simulink model "STM_sim"  (R2024b)
settings: Solver=ode3  StartTime=0.0  StopTime=time_simulated  FixedStep=time_step_size  RelTol=1e-3
values from neighbouring files (symbols this model uses):
  a = 0.276626506024    [Fufy.mat]    (also in STMDrift.m = 1.347; Trajectory_LQR_double_track_Workspace_Phase_Plane_16_06.m = l-b; initParam.m = l-b)
  b = 0.283373493976    [Fufy.mat]    (also in STMDrift.m = 1.393; Trajectory_LQR_double_track_Workspace_Phase_Plane_16_06.m = l/2; initParam.m = l/2)
  constant_force = 9    [runSIM.m]
  constant_steer = deg2rad(15)    [runSIM.m]
  Fz_Front_nominal = Fz_Front    [initParam.m]
  Fz_Rear_nominal = Fz_Rear    [initParam.m]
  gamma = pi/2    (= 1.57079632679)    [Trajectory_LQR_double_track_Workspace_Phase_Plane_16_06.m]    (also in initParam.m)
  J_CoG = 1.30125108434    [Fufy.mat]    (also in Trajectory_LQR_double_track_Workspace_Phase_Plane_16_06.m = 9.4*a^2+9.4*b^2; initParam.m = 9.4*a^2+9.4*b^2)
  m = 16.6    [Fufy.mat]    (also in STMDrift.m = 2137.3; Trajectory_LQR_double_track_Workspace_Phase_Plane_16_06.m = 18.8; initParam.m = 18.8)
  steering_ratio_f = 0.6    [Fufy.mat]
  t_front = t    [Trajectory_LQR_double_track_Workspace_Phase_Plane_16_06.m]    (also in initParam.m)
  t_rear = t    [Trajectory_LQR_double_track_Workspace_Phase_Plane_16_06.m]    (also in initParam.m)
  u0 = 0    [Trajectory_LQR_double_track_Workspace_Phase_Plane_16_06.m]    (also in runSIM.m)
  v0 = 0    [Trajectory_LQR_double_track_Workspace_Phase_Plane_16_06.m]    (also in runSIM.m)
  x0 = 0    [Trajectory_LQR_double_track_Workspace_Phase_Plane_16_06.m]    (also in initParam.m)
  y0 = 0    [Trajectory_LQR_double_track_Workspace_Phase_Plane_16_06.m]    (also in initParam.m)
  yaw_rate0 = 0    [Trajectory_LQR_double_track_Workspace_Phase_Plane_16_06.m]    (also in runSIM.m)
settings Model: Creator=pc  LastModifiedBy=mg

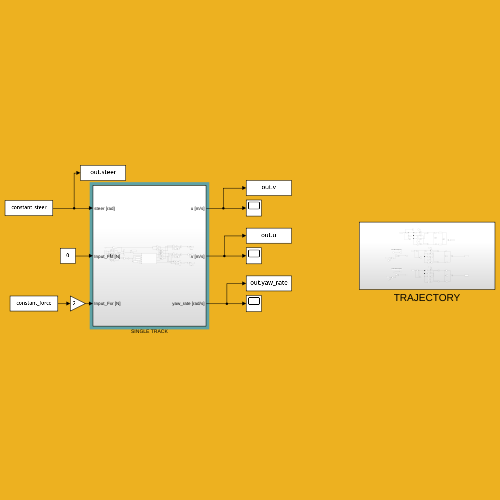
[thumbnail: Simulink's stored preview of the top-level diagram]
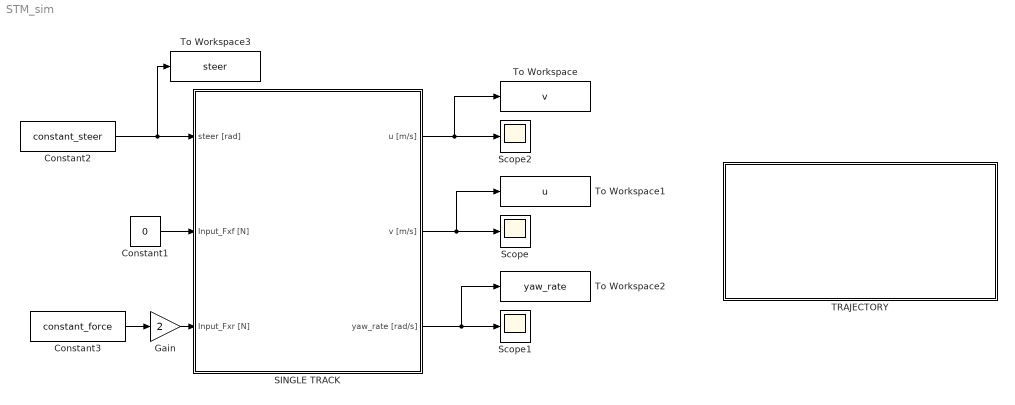
== system STM_sim ==
  Constant1 : Constant  Value=0
  Constant2 : Constant  Value=constant_steer
  Constant3 : Constant  Value=constant_force
  Gain : Gain  Gain=2
  SINGLE TRACK : Subsystem
  Scope : Scope
  Scope1 : Scope
  Scope2 : Scope
  TRAJECTORY : Subsystem
  To Workspace : ToWorkspace  VariableName=v  SampleTime=-1
  To Workspace1 : ToWorkspace  VariableName=u  SampleTime=-1
  To Workspace2 : ToWorkspace  VariableName=yaw_rate  SampleTime=-1
  To Workspace3 : ToWorkspace  VariableName=steer  SampleTime=-1
  wires:
  Constant1/1 -> SINGLE TRACK/2(Input_Fxf [N])
  Constant2/1 -> To Workspace3/1, SINGLE TRACK/1(steer [rad])
  SINGLE TRACK/2(v [m/s]) -> Scope/1, To Workspace1/1
  SINGLE TRACK/3(yaw_rate [rad/s]) -> Scope1/1, To Workspace2/1
  SINGLE TRACK/1(u [m/s]) -> Scope2/1, To Workspace/1
  Gain/1 -> SINGLE TRACK/3(Input_Fxr [N])
  Constant3/1 -> Gain/1

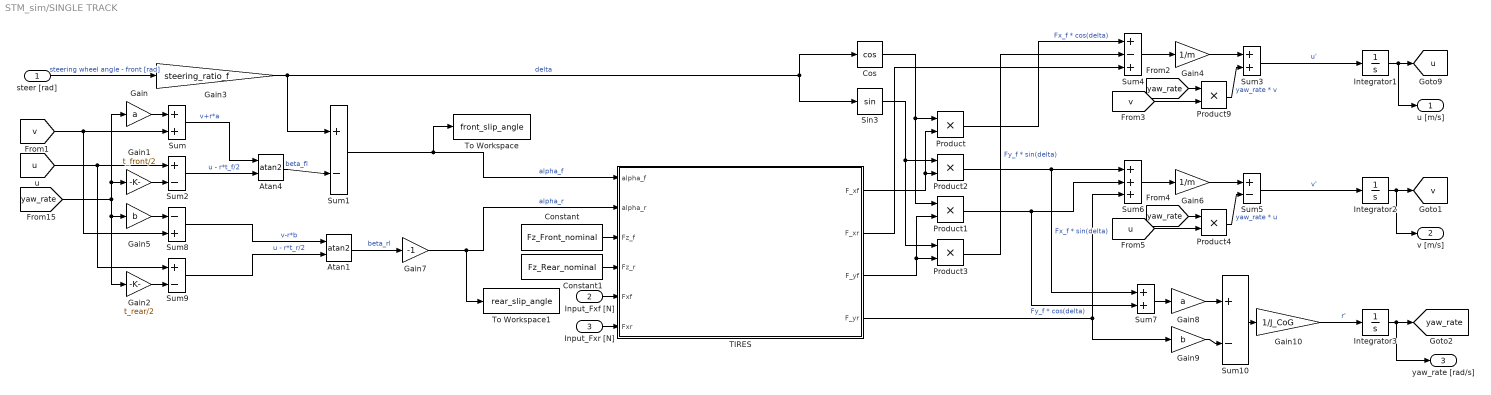
== system STM_sim/SINGLE TRACK ==
  steer [rad] : Inport
  Input_Fxf [N] : Inport  Port=2
  Input_Fxr [N] : Inport  Port=3
  Atan1 : Trigonometry  Operator=atan2
  Atan4 : Trigonometry  Operator=atan2
  Constant : Constant  Value=Fz_Front_nominal
  Constant1 : Constant  Value=Fz_Rear_nominal
  Cos : Trigonometry  Operator=cos
  Gain : Gain  Gain=a
  Gain1 : Gain  Gain=t_front/2
  Gain10 : Gain  Gain=1/J_CoG
  Gain2 : Gain  Gain=t_rear/2
  Gain3 : Gain  Gain=steering_ratio_f
  Gain4 : Gain  Gain=1/m
  Gain5 : Gain  Gain=b
  Gain6 : Gain  Gain=1/m
  Gain7 : Gain  Gain=-1
  Gain8 : Gain  Gain=a
  Gain9 : Gain  Gain=b
  Integrator1 : Integrator  InitialCondition=u0
  Integrator2 : Integrator  InitialCondition=v0
  Integrator3 : Integrator  InitialCondition=yaw_rate0
  Product{,1..4,9} (6 alike) : Product
  Sin3 : Trigonometry
  Sum : Sum  Inputs=||+|||+||
  Sum1 : Sum  Inputs=||+||-||
  Sum10 : Sum  Inputs=||+||-||
  Sum2 : Sum  Inputs=||+|||-||
  Sum3 : Sum  Inputs=||+||+||
  Sum4 : Sum  Inputs=||+||-||+||
  Sum5 : Sum  Inputs=||+||-||
  Sum6 : Sum  Inputs=||+||+||+||
  Sum7 : Sum  Inputs=||+||+||
  Sum8 : Sum  Inputs=||-|||+||
  Sum9 : Sum  Inputs=||+|||-||
  TIRES : MATLAB Function  TreatAsAtomicUnit=on
  To Workspace : ToWorkspace  VariableName=front_slip_angle  SampleTime=-1
  To Workspace1 : ToWorkspace  VariableName=rear_slip_angle  SampleTime=-1
  u [m/s] : Outport
  v [m/s] : Outport  Port=2
  yaw_rate [rad/s] : Outport  Port=3
  tag scope: u=global, v=global, yaw_rate=global
  wires:
  Integrator3/1 -> [yaw_rate], yaw_rate [rad/s]/1
  Integrator2/1 -> [v], v [m/s]/1
  Integrator1/1 -> [u], u [m/s]/1
  Gain10/1 -> Integrator3/1  "r'"
  Sum10/1 -> Gain10/1
  Gain9/1 -> Sum10/2
  Gain8/1 -> Sum10/1
  Sum7/1 -> Gain8/1
  Sum6/1 -> Gain6/1
  Product4/1 -> Sum5/2  "yaw_rate * u"
  [u] -> Product4/2
  [yaw_rate] -> Product4/1
  Sum5/1 -> Integrator2/1  "v'"
  Gain6/1 -> Sum5/1
  [v] -> Product9/2
  Product9/1 -> Sum3/2  "yaw_rate * v"
  [yaw_rate] -> Product9/1
  Sum3/1 -> Integrator1/1  "u'"
  Gain4/1 -> Sum3/1
  Sum4/1 -> Gain4/1
  Product3/1 -> Sum4/2  "Fy_f * sin(delta)"
  Product2/1 -> Sum6/1, Sum7/1  "Fx_f * sin(delta)"
  Product/1 -> Sum4/1  "Fx_f * cos(delta)"
  Product1/1 -> Sum7/2, Sum6/2  "Fy_f * cos(delta)"
  Sin3/1 -> Product2/1, Product3/1
  Cos/1 -> Product/1, Product1/1
  TIRES/4(F_yr) -> Gain9/1, Sum6/3
  Constant/1 -> TIRES/3(Fz_f)
  Input_Fxf [N]/1 -> TIRES/5(Fxf)
  Gain5/1 -> Sum8/1
  steer [rad]/1 -> Gain3/1  "steering wheel angle - front [rad]"
  TIRES/2(F_xr) -> Sum4/3
  Sum2/1 -> Atan4/2  "u - r*t_f/2"
  Constant1/1 -> TIRES/4(Fz_r)
  Gain3/1 -> Sin3/1, Cos/1, Sum1/1  "delta"
  Sum/1 -> Atan4/1  "v+r*a"
  [yaw_rate] -> Gain5/1, Gain2/1, Gain1/1, Gain/1
  [v] -> Sum/2, Sum8/2
  Gain2/1 -> Sum9/2
  [u] -> Sum2/1, Sum9/1
  TIRES/3(F_yf) -> Product1/2, Product3/2
  TIRES/1(F_xf) -> Product/2, Product2/2
  Atan4/1 -> Sum1/2  "beta_fl"
  Sum8/1 -> Atan1/1  "v-r*b"
  Gain/1 -> Sum/1
  Gain7/1 -> TIRES/2(alpha_r), To Workspace1/1  "alpha_r"
  Input_Fxr [N]/1 -> TIRES/6(Fxr)
  Sum9/1 -> Atan1/2  "u - r*t_r/2"
  Gain1/1 -> Sum2/2
  Atan1/1 -> Gain7/1  "beta_rl"
  Sum1/1 -> TIRES/1(alpha_f), To Workspace/1  "alpha_f"

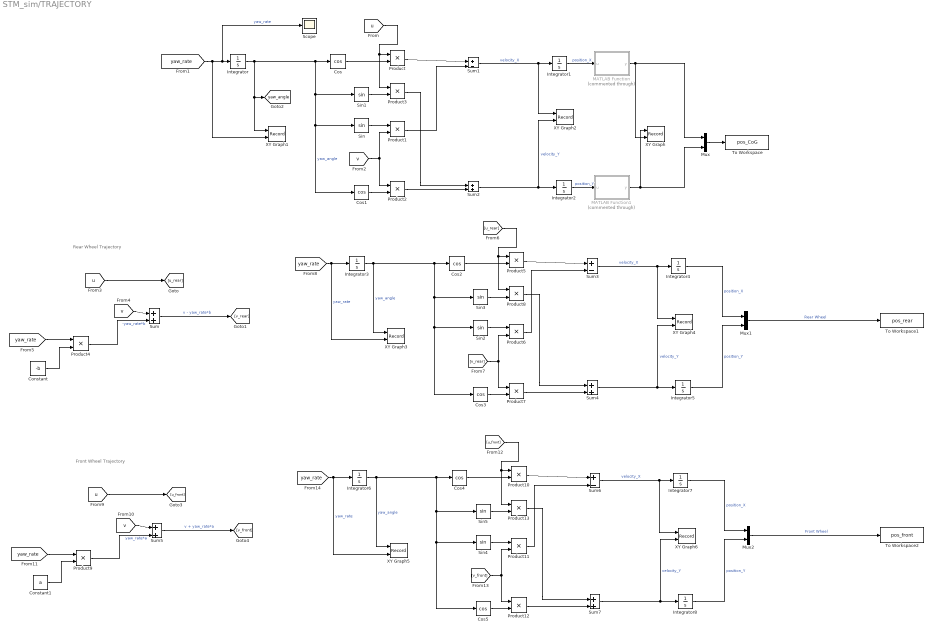
== system STM_sim/TRAJECTORY ==
  note: Front Wheel Trajectory
  note: Rear Wheel Trajectory
  Constant : Constant  Value=-b
  Constant1 : Constant  Value=a
  Cos{,1..5} (6 alike) : Trigonometry  Operator=cos
  Integrator : Integrator  InitialCondition=gamma
  Integrator1 : Integrator  InitialCondition=x0
  Integrator2 : Integrator  InitialCondition=y0
  Integrator3 : Integrator  InitialCondition=gamma
  Integrator4 : Integrator  InitialCondition=x0
  Integrator5 : Integrator  InitialCondition=y0-b
  Integrator6 : Integrator  InitialCondition=gamma
  Integrator7 : Integrator  InitialCondition=x0
  Integrator8 : Integrator  InitialCondition=y0+a
  MATLAB Function : MATLAB Function  Commented=through  TreatAsAtomicUnit=on
  MATLAB Function1 : MATLAB Function  Commented=through  TreatAsAtomicUnit=on
  Mux : Mux  Inputs=2
  Mux1 : Mux  Inputs=2
  Mux2 : Mux  Inputs=2
  Product{,1..13} (14 alike) : Product
  Scope : Scope
  Sin{,1..5} (6 alike) : Trigonometry
  Sum{,4..5,7} (4 alike) : Sum  Inputs=|+|||+|
  Sum1 : Sum  Inputs=+||-
  Sum2 : Sum  Inputs=+||+
  Sum3 : Sum  Inputs=|+|||-|
  Sum6 : Sum  Inputs=|+|||-|
  To Workspace : ToWorkspace  VariableName=pos_CoG  SampleTime=-1
  To Workspace1 : ToWorkspace  VariableName=pos_rear  SampleTime=-1
  To Workspace2 : ToWorkspace  VariableName=pos_front  SampleTime=-1
  XY Graph : Record  FileSettingsInternal="{\"entries\":[{\"content\":{\"excelSettings\":{\"content\":{},\"type\":\"Streamout.ExcelSettings\"}},\"type\":\"Streamout.FileSettingStorage\",\"uuid\":\"\"}],\"packageUris\":[\"http:\\/\\/schema.mathworks.com\\/mf0\\/streamout_blocks\\/R2020a\"],\"version\":\"1.0\"}"  Layout=[1 1]  SignalsInternal="{\"entries\":[{\"content\":{\"signals\":[{\"content\":{\"blockPath\":[],\"dimensions\":[1],\"domain\":\"\",\"lineColor\":\"#b746ff\",\"lineWidth\":2,\"port\":1,\"sid\":[\"\"],\"signalID\":1,\"signalName\":\"MATLAB Function1\"},\"type\":\"RecordBlkView.Signal\",\"uuid\":\"\"},{\"content\":{\"blockPath\":[],\"dimensions\":[1],\"domain\":\"\",\"lineColor\":\"#64d413\",\"lineWidth\":2,\"port\":2,\"sid\":[\"\"],\"signalID\":2,\"signalName\":\"MATLAB Function\"},\"type\":\"RecordBlkView.Signal\",\"uuid\":\"\"}]},\"type\":\"RecordBlkView.InputSignals\",\"uuid\":\"\"}],\"packageUris\":[\"http:\\/\\/schema.mathworks.com\\/mf0\\/streamout_blocks\\/R2020a\"],\"version\":\"1.0\"}"  VisualizationBindings="{\"xyplotplugin\":{\"info\":[{\"series\":[],\"subplotID\":1}]}}"  CompatibilityTag=XY
  XY Graph1 : Record  FileSettingsInternal="{\"entries\":[{\"content\":{\"excelSettings\":{\"content\":{},\"type\":\"Streamout.ExcelSettings\"}},\"type\":\"Streamout.FileSettingStorage\",\"uuid\":\"\"}],\"packageUris\":[\"http:\\/\\/schema.mathworks.com\\/mf0\\/streamout_blocks\\/R2020a\"],\"version\":\"1.0\"}"  Layout=[1 1]  SignalsInternal="{\"entries\":[{\"content\":{\"signals\":[{\"content\":{\"blockPath\":[],\"dimensions\":[1],\"domain\":\"\",\"lineColor\":\"#ff13a6\",\"lineWidth\":2,\"port\":1,\"sid\":[\"\"],\"signalID\":1,\"signalName\":\"yaw_angle\"},\"type\":\"RecordBlkView.Signal\",\"uuid\":\"\"},{\"content\":{\"blockPath\":[],\"dimensions\":[1],\"domain\":\"\",\"lineColor\":\"#fe330a\",\"lineWidth\":2,\"port\":2,\"sid\":[\"\"],\"signalID\":2,\"signalName\":\"yaw_rate\"},\"type\":\"RecordBlkView.Signal\",\"uuid\":\"\"}]},\"type\":\"RecordBlkView.InputSignals\",\"uuid\":\"\"}],\"packageUris\":[\"http:\\/\\/schema.mathworks.com\\/mf0\\/streamout_blocks\\/R2020a\"],\"version\":\"1.0\"}"  VisualizationBindings="{\"sparklinesplugin\":{\"info\":[{\"bindingParametersList\":[],\"subplotID\":1}]}}"  CompatibilityTag=XY
  XY Graph2 : Record  FileSettingsInternal="{\"entries\":[{\"content\":{\"excelSettings\":{\"content\":{},\"type\":\"Streamout.ExcelSettings\"}},\"type\":\"Streamout.FileSettingStorage\",\"uuid\":\"\"}],\"packageUris\":[\"http:\\/\\/schema.mathworks.com\\/mf0\\/streamout_blocks\\/R2020a\"],\"version\":\"1.0\"}"  Layout=[1 1]  SignalsInternal="{\"entries\":[{\"content\":{\"signals\":[{\"content\":{\"blockPath\":[],\"dimensions\":[1],\"domain\":\"\",\"lineColor\":\"#22b573\",\"lineWidth\":2,\"port\":1,\"sid\":[\"\"],\"signalID\":1,\"signalName\":\"velocity_X\"},\"type\":\"RecordBlkView.Signal\",\"uuid\":\"\"},{\"content\":{\"blockPath\":[],\"dimensions\":[1],\"domain\":\"\",\"lineColor\":\"#0072bd\",\"lineWidth\":2,\"port\":2,\"sid\":[\"\"],\"signalID\":2,\"signalName\":\"velocity_Y\"},\"type\":\"RecordBlkView.Signal\",\"uuid\":\"\"}]},\"type\":\"RecordBlkView.InputSignals\",\"uuid\":\"\"}],\"packageUris\":[\"http:\\/\\/schema.mathworks.com\\/mf0\\/streamout_blocks\\/R2020a\"],\"version\":\"1.0\"}"  VisualizationBindings="{\"sparklinesplugin\":{\"info\":[{\"bindingParametersList\":[],\"subplotID\":1}]}}"  CompatibilityTag=XY
  XY Graph3 : Record  FileSettingsInternal="{\"entries\":[{\"content\":{\"excelSettings\":{\"content\":{},\"type\":\"Streamout.ExcelSettings\"}},\"type\":\"Streamout.FileSettingStorage\",\"uuid\":\"\"}],\"packageUris\":[\"http:\\/\\/schema.mathworks.com\\/mf0\\/streamout_blocks\\/R2020a\"],\"version\":\"1.0\"}"  Layout=[1 1]  SignalsInternal="{\"entries\":[{\"content\":{\"signals\":[{\"content\":{\"blockPath\":[],\"dimensions\":[1],\"domain\":\"\",\"lineColor\":\"#ff13a6\",\"lineWidth\":2,\"port\":1,\"sid\":[\"\"],\"signalID\":1,\"signalName\":\"yaw_angle\"},\"type\":\"RecordBlkView.Signal\",\"uuid\":\"\"},{\"content\":{\"blockPath\":[],\"dimensions\":[1],\"domain\":\"\",\"lineColor\":\"#fe330a\",\"lineWidth\":2,\"port\":2,\"sid\":[\"\"],\"signalID\":2,\"signalName\":\"yaw_rate\"},\"type\":\"RecordBlkView.Signal\",\"uuid\":\"\"}]},\"type\":\"RecordBlkView.InputSignals\",\"uuid\":\"\"}],\"packageUris\":[\"http:\\/\\/schema.mathworks.com\\/mf0\\/streamout_blocks\\/R2020a\"],\"version\":\"1.0\"}"  VisualizationBindings="{\"sparklinesplugin\":{\"info\":[{\"bindingParametersList\":[],\"subplotID\":1}]}}"  CompatibilityTag=XY
  XY Graph4 : Record  FileSettingsInternal="{\"entries\":[{\"content\":{\"excelSettings\":{\"content\":{},\"type\":\"Streamout.ExcelSettings\"}},\"type\":\"Streamout.FileSettingStorage\",\"uuid\":\"\"}],\"packageUris\":[\"http:\\/\\/schema.mathworks.com\\/mf0\\/streamout_blocks\\/R2020a\"],\"version\":\"1.0\"}"  Layout=[1 1]  SignalsInternal="{\"entries\":[{\"content\":{\"signals\":[{\"content\":{\"blockPath\":[],\"dimensions\":[1],\"domain\":\"\",\"lineColor\":\"#22b573\",\"lineWidth\":2,\"port\":1,\"sid\":[\"\"],\"signalID\":1,\"signalName\":\"velocity_X\"},\"type\":\"RecordBlkView.Signal\",\"uuid\":\"\"},{\"content\":{\"blockPath\":[],\"dimensions\":[1],\"domain\":\"\",\"lineColor\":\"#0072bd\",\"lineWidth\":2,\"port\":2,\"sid\":[\"\"],\"signalID\":2,\"signalName\":\"velocity_Y\"},\"type\":\"RecordBlkView.Signal\",\"uuid\":\"\"}]},\"type\":\"RecordBlkView.InputSignals\",\"uuid\":\"\"}],\"packageUris\":[\"http:\\/\\/schema.mathworks.com\\/mf0\\/streamout_blocks\\/R2020a\"],\"version\":\"1.0\"}"  VisualizationBindings="{\"sparklinesplugin\":{\"info\":[{\"bindingParametersList\":[],\"subplotID\":1}]}}"  CompatibilityTag=XY
  XY Graph5 : Record  FileSettingsInternal="{\"entries\":[{\"content\":{\"excelSettings\":{\"content\":{},\"type\":\"Streamout.ExcelSettings\"}},\"type\":\"Streamout.FileSettingStorage\",\"uuid\":\"\"}],\"packageUris\":[\"http:\\/\\/schema.mathworks.com\\/mf0\\/streamout_blocks\\/R2020a\"],\"version\":\"1.0\"}"  Layout=[1 1]  SignalsInternal="{\"entries\":[{\"content\":{\"signals\":[{\"content\":{\"blockPath\":[],\"dimensions\":[1],\"domain\":\"\",\"lineColor\":\"#7e2f8e\",\"lineWidth\":2,\"port\":1,\"sid\":[\"\"],\"signalID\":1,\"signalName\":\"yaw_angle\"},\"type\":\"RecordBlkView.Signal\",\"uuid\":\"\"},{\"content\":{\"blockPath\":[],\"dimensions\":[1],\"domain\":\"\",\"lineColor\":\"#77ac30\",\"lineWidth\":2,\"port\":2,\"sid\":[\"\"],\"signalID\":2,\"signalName\":\"yaw_rate\"},\"type\":\"RecordBlkView.Signal\",\"uuid\":\"\"}]},\"type\":\"RecordBlkView.InputSignals\",\"uuid\":\"\"}],\"packageUris\":[\"http:\\/\\/schema.mathworks.com\\/mf0\\/streamout_blocks\\/R2020a\"],\"version\":\"1.0\"}"  VisualizationBindings="{\"sparklinesplugin\":{\"info\":[{\"bindingParametersList\":[],\"subplotID\":1}]}}"  CompatibilityTag=XY
  XY Graph6 : Record  FileSettingsInternal="{\"entries\":[{\"content\":{\"excelSettings\":{\"content\":{},\"type\":\"Streamout.ExcelSettings\"}},\"type\":\"Streamout.FileSettingStorage\",\"uuid\":\"\"}],\"packageUris\":[\"http:\\/\\/schema.mathworks.com\\/mf0\\/streamout_blocks\\/R2020a\"],\"version\":\"1.0\"}"  Layout=[1 1]  SignalsInternal="{\"entries\":[{\"content\":{\"signals\":[{\"content\":{\"blockPath\":[],\"dimensions\":[1],\"domain\":\"\",\"lineColor\":\"#4dbeee\",\"lineWidth\":2,\"port\":1,\"sid\":[\"\"],\"signalID\":1,\"signalName\":\"velocity_X\"},\"type\":\"RecordBlkView.Signal\",\"uuid\":\"\"},{\"content\":{\"blockPath\":[],\"dimensions\":[1],\"domain\":\"\",\"lineColor\":\"#a2142f\",\"lineWidth\":2,\"port\":2,\"sid\":[\"\"],\"signalID\":2,\"signalName\":\"velocity_Y\"},\"type\":\"RecordBlkView.Signal\",\"uuid\":\"\"}]},\"type\":\"RecordBlkView.InputSignals\",\"uuid\":\"\"}],\"packageUris\":[\"http:\\/\\/schema.mathworks.com\\/mf0\\/streamout_blocks\\/R2020a\"],\"version\":\"1.0\"}"  VisualizationBindings="{\"sparklinesplugin\":{\"info\":[{\"bindingParametersList\":[],\"subplotID\":1}]}}"  CompatibilityTag=XY
  tag scope: yaw_angle=global
  wires:
  Mux/1 -> To Workspace/1
  Product4/1 -> Sum/2  "-yaw_rate*b"
  Integrator3/1 -> XY Graph3/1, Cos2/1, Sin3/1, Sin2/1, Cos3/1  "yaw_angle"
  Product10/1 -> Sum6/1
  Mux1/1 -> To Workspace1/1  "Rear Wheel"
  Mux2/1 -> To Workspace2/1  "Front Wheel"
  Sum/1 -> [v_rear]  "v - yaw_rate*b"
  Integrator8/1 -> Mux2/2  "position_Y"
  Product6/1 -> Sum3/2
  Cos5/1 -> Product12/2
  Product5/1 -> Sum3/1
  Integrator4/1 -> Mux1/1  "position_X"
  Constant/1 -> Product4/2
  [v] -> Sum/1
  Sin3/1 -> Product8/2
  Sum3/1 -> Integrator4/1, XY Graph4/1  "velocity_X"
  Product11/1 -> Sum6/2
  Cos3/1 -> Product7/2
  [yaw_rate] -> Product4/1
  Sum4/1 -> XY Graph4/2, Integrator5/1  "velocity_Y"
  Cos2/1 -> Product5/2
  Sum7/1 -> XY Graph6/2, Integrator8/1  "velocity_Y"
  Sin2/1 -> Product6/1
  [u] -> [u_rear]
  Product8/1 -> Sum4/1
  [v] -> Sum5/1
  Sin4/1 -> Product11/1
  [yaw_rate] -> Integrator3/1, XY Graph3/2  "yaw_rate"
  Product9/1 -> Sum5/2  "yaw_rate*a"
  Integrator6/1 -> XY Graph5/1, Cos4/1, Sin5/1, Sin4/1, Cos5/1  "yaw_angle"
  [v_front] -> Product12/1, Product11/2
  Product7/1 -> Sum4/2
  Integrator5/1 -> Mux1/2  "position_Y"
  Product12/1 -> Sum7/2
  [u] -> [u_front]
  [yaw_rate] -> Integrator6/1, XY Graph5/2  "yaw_rate"
  [v_rear] -> Product7/1, Product6/2
  [u_front] -> Product10/1, Product13/1
  Sum6/1 -> Integrator7/1, XY Graph6/1  "velocity_X"
  [u_rear] -> Product5/1, Product8/1
  Sum5/1 -> [v_front]  "v + yaw_rate*a"
  Integrator7/1 -> Mux2/1  "position_X"
  Constant1/1 -> Product9/2
  Cos4/1 -> Product10/2
  Sin5/1 -> Product13/2
  [yaw_rate] -> Product9/1
  Product13/1 -> Sum7/1
  MATLAB Function1/1(y) -> XY Graph/1, Mux/2
  MATLAB Function/1(y) -> XY Graph/2, Mux/1
  Integrator1/1 -> MATLAB Function/1(u)  "position_X"
  Integrator/1 -> XY Graph1/1, [yaw_angle], Cos/1, Sin1/1, Sin/1, Cos1/1  "yaw_angle"
  Sin1/1 -> Product3/2
  Product1/1 -> Sum1/2
  [v] -> Product2/1, Product1/2
  Sin/1 -> Product1/1
  [yaw_rate] -> Integrator/1, Scope/1, XY Graph1/2  "yaw_rate"
  Cos/1 -> Product/2
  Sum1/1 -> Integrator1/1, XY Graph2/1  "velocity_X"
  [u] -> Product/1, Product3/1
  Sum2/1 -> Integrator2/1, XY Graph2/2  "velocity_Y"
  Product/1 -> Sum1/1
  Product2/1 -> Sum2/2
  Cos1/1 -> Product2/2
  Integrator2/1 -> MATLAB Function1/1(u)  "position_Y"
  Product3/1 -> Sum2/1

== matlab function STM_sim/TRAJECTORY/MATLAB Function ==
  data: u input; y output
function y = fcn(u)
n = 3;
    %#codegen
    y = round(u * 10^n) / 10^n;
end

== matlab function STM_sim/TRAJECTORY/MATLAB Function1 ==
  data: u input; y output
function y = fcn(u)
n = 3;
    %#codegen
    y = round(u * 10^n) / 10^n;
end

== matlab function STM_sim/SINGLE TRACK/TIRES ==
  data: alpha_f input; alpha_r input; Fz_f input; Fz_r input; Fxf input; Fxr input; F_xf output; F_xr output; F_yf output; F_yr output
function [F_xf,F_xr,F_yf,F_yr] = fcn(alpha_f,alpha_r,Fz_f,Fz_r,Fxf,Fxr) 
%% Separation of inputs variable
% alpha_fl = inputs(1); % [rad]
% alpha_rl  = inputs(2); % [rad]
% Fz_f = inputs(3); % [N] vertical load on front axle
% Fz_r = inputs(4); % [N] vertical load on rear axle
% Fxf = inputs(5); % [N] longitudinal left frontal force
% Fxr  = inputs(6); % [N] longitudinal left rear force

%% Maximum saturation and Stiffness
F_ymax = @(mu,Fz,Fx) sqrt((mu*Fz)^2-Fx^2);

alpha_s= @(Fy_max,C_alpha) atan((3*Fy_max)/C_alpha); % [rad] maximum slip angle beyond which tire starts to slide

Cy_front  = 370.36; %[N/rad] Cornering stiffness front tyre
Cy_rear   = 1134.05;%[N/rad] Cornering stiffness rear tyre

mu_front  = 0.5;
mu_rear   = 0.47;

%% Longitudinal forces 

F_xf = Fxf; % [N] 
F_xr = Fxr; % [N] 

% saturation of the tire
if abs(F_xr) > mu_rear*Fz_r - 0.0001
    F_xr = (mu_rear*Fz_r - 0.0001)*sign(F_xr);
end

F_ymaxrear = F_ymax(mu_rear,Fz_r,F_xr);
F_ymaxfront = F_ymax(mu_front,Fz_f,F_xf);

%% Lateral forces 
Fy_fiala = @(Fy_max,Cy,mu,alpha) Cy*tan(alpha)- ...
                                        Cy^2./(3*Fy_max).*abs(tan(alpha)).*tan(alpha)+ ...
                                        Cy^3./(27*(Fy_max)^2).*(tan(alpha)).^3; 


%________ FRONT
if abs(alpha_f) >= alpha_s(F_ymaxfront,Cy_front)
    F_yf = F_ymaxfront*sign(alpha_f);
else
    F_yf = Fy_fiala(F_ymaxfront,Cy_front,mu_front,abs(alpha_f))*sign(alpha_f);
end

%________ REAR
if abs(alpha_r) >= alpha_s(F_ymaxrear,Cy_rear)
    F_yr = F_ymaxrear*sign(alpha_r);
else
    F_yr = Fy_fiala(F_ymaxrear,Cy_rear,mu_rear,abs(alpha_r))*sign(alpha_r);
end
